simulink subsystem "rss_foc_controller_NewPlatform"  (R2023a)
settings: Solver=VariableStepAuto  StartTime=0.0  StopTime=10.0  RelTol=1e-3
undefined symbols (not defined in the file): Cdbl_tiFstTaskSmpTi, Cdbl_tiMedTaskSmpTi, Cdbl_tiSlwTaskSmpTi, ENM_AG_POS_EVAL_MODE, ENM_MOTO_STATUS, ENM_SYS_STATUS
(part 2 of 2)

== system rss_foc_controller_NewPlatform/vrs_DcycGenFstTaskIn/sss_DcycGenFstTaskInSenl ==
  u16_ampDycAmp : Inport
  u16_phiActElecAg : Inport  Port=2
  u16_phiDaxQaxVltgAg : Inport  Port=3
  enm_stMotoSt : Inport  Port=4
  s16_nPredActElecSpd : Inport  Port=5
  Bus Creator : BusCreator  Inputs=5  OutDataTypeStr=Bus: BUS_DCYCGEN_FST_TASK_IN
      settings: InheritFromInputs=off
  busDcycGen_FstTaskIn : Outport
  wires:
  Bus Creator/1 -> busDcycGen_FstTaskIn/1
  u16_ampDycAmp/1 -> Bus Creator/1
  u16_phiDaxQaxVltgAg/1 -> Bus Creator/3
  u16_phiActElecAg/1 -> Bus Creator/2
  s16_nPredActElecSpd/1 -> Bus Creator/5
  enm_stMotoSt/1 -> Bus Creator/4

== system rss_foc_controller_NewPlatform/vrs_DcycGenFstTaskIn/sss_DcycGenFstTaskInSens ==
  u16_ampDycAmp : Inport
  u16_phiActElecAg : Inport  Port=2
  u16_phiDaxQaxVltgAg : Inport  Port=3
  enm_stMotoSt : Inport  Port=4
  s16_nPredActElecSpd : Inport  Port=5
  bol_enPosSCDCalibEnFlg : Inport  Port=6
  Bus Creator : BusCreator  Inputs=6  OutDataTypeStr=Bus: BUS_DCYCGEN_FST_TASK_IN
      settings: InheritFromInputs=off
  busDcycGen_FstTaskIn : Outport
  wires:
  Bus Creator/1 -> busDcycGen_FstTaskIn/1
  bol_enPosSCDCalibEnFlg/1 -> Bus Creator/6
  u16_ampDycAmp/1 -> Bus Creator/1
  u16_phiDaxQaxVltgAg/1 -> Bus Creator/3
  u16_phiActElecAg/1 -> Bus Creator/2
  s16_nPredActElecSpd/1 -> Bus Creator/5
  enm_stMotoSt/1 -> Bus Creator/4

== system rss_foc_controller_NewPlatform/vrs_DcycGenFstTaskOut/sss_DcycGenFstTaskOutSenl ==
  busDcycGen_FstTaskOut : Inport
  Bus Selector1 : BusSelector  OutputSignals=u16_dcycPhDyc,u16_ampMaxNrmVltgAmp,u16_phiModulActElecAg
  u16_dcycPhDyc : Outport
  u16_ampMaxNrmVltgAmp : Outport  Port=2
  u16_phiModulActElecAg : Outport  Port=3
  wires:
  Bus Selector1/3 -> u16_phiModulActElecAg/1  "<u16_phiModulActElecAg>"
  Bus Selector1/1 -> u16_dcycPhDyc/1  "<u16_dcycPhDyc>"
  busDcycGen_FstTaskOut/1 -> Bus Selector1/1
  Bus Selector1/2 -> u16_ampMaxNrmVltgAmp/1  "<u16_ampMaxNrmVltgAmp>"

== system rss_foc_controller_NewPlatform/vrs_DcycGenFstTaskOut/sss_DcycGenFstTaskOutSens ==
  busDcycGen_FstTaskOut : Inport
  Bus Selector1 : BusSelector  OutputSignals=u16_dcycPhDyc,u16_ampMaxNrmVltgAmp,u16_phiModulActElecAg
  u16_dcycPhDyc : Outport
  u16_ampMaxNrmVltgAmp : Outport  Port=2
  u16_phiModulActElecAg : Outport  Port=3
  wires:
  Bus Selector1/3 -> u16_phiModulActElecAg/1  "<u16_phiModulActElecAg>"
  Bus Selector1/1 -> u16_dcycPhDyc/1  "<u16_dcycPhDyc>"
  busDcycGen_FstTaskOut/1 -> Bus Selector1/1
  Bus Selector1/2 -> u16_ampMaxNrmVltgAmp/1  "<u16_ampMaxNrmVltgAmp>"

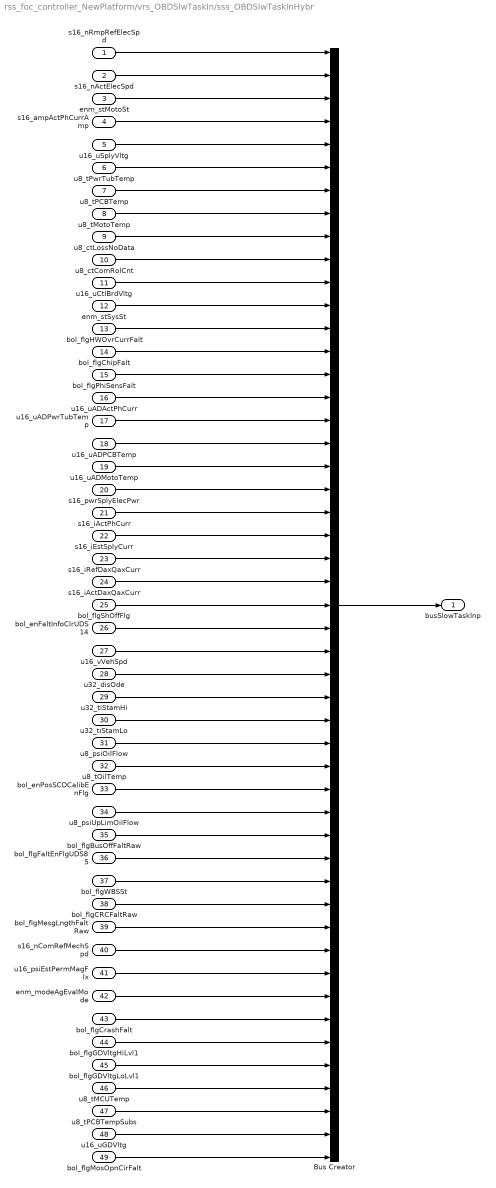
== system rss_foc_controller_NewPlatform/vrs_OBDSlwTaskIn/sss_OBDSlwTaskInHybr ==
  s16_nRmpRefElecSpd : Inport
  s16_nActElecSpd : Inport  Port=2
  enm_stMotoSt : Inport  Port=3
  s16_ampActPhCurrAmp : Inport  Port=4
  u16_uSplyVltg : Inport  Port=5
  u8_tPwrTubTemp : Inport  Port=6
  u8_tPCBTemp : Inport  Port=7
  u8_tMotoTemp : Inport  Port=8
  u8_ctLossNoData : Inport  Port=9
  u8_ctComRolCnt : Inport  Port=10
  u16_uCtlBrdVltg : Inport  Port=11
  enm_stSysSt : Inport  Port=12
  bol_flgHWOvrCurrFalt : Inport  Port=13
  bol_flgChipFalt : Inport  Port=14
  bol_flgPhiSensFalt : Inport  Port=15
  u16_uADActPhCurr : Inport  Port=16
  u16_uADPwrTubTemp : Inport  Port=17
  u16_uADPCBTemp : Inport  Port=18
  u16_uADMotoTemp : Inport  Port=19
  s16_pwrSplyElecPwr : Inport  Port=20
  s16_iActPhCurr : Inport  Port=21
  s16_iEstSplyCurr : Inport  Port=22
  s16_iRefDaxQaxCurr : Inport  Port=23
  s16_iActDaxQaxCurr : Inport  Port=24
  bol_flgShOffFlg : Inport  Port=25
  bol_enFaltInfoClrUDS14 : Inport  Port=26
  u16_vVehSpd : Inport  Port=27
  u32_disOde : Inport  Port=28
  u32_tiStamHi : Inport  Port=29
  u32_tiStamLo : Inport  Port=30
  u8_psiOilFlow : Inport  Port=31
  u8_tOilTemp : Inport  Port=32
  bol_enPosSCDCalibEnFlg : Inport  Port=33
  u8_psiUpLimOilFlow : Inport  Port=34
  bol_flgBusOffFaltRaw : Inport  Port=35
  bol_flgFaltEnFlgUDS85 : Inport  Port=36
  bol_flgWBSSt : Inport  Port=37
  bol_flgCRCFaltRaw : Inport  Port=38
  bol_flgMesgLngthFaltRaw : Inport  Port=39
  s16_nComRefMechSpd : Inport  Port=40
  u16_psiEstPermMagFlx : Inport  Port=41
  enm_modeAgEvalMode : Inport  Port=42
  bol_flgCrashFalt : Inport  Port=43
  bol_flgGDVltgHiLvl1 : Inport  Port=44
  bol_flgGDVltgLoLvl1 : Inport  Port=45
  u8_tMCUTemp : Inport  Port=46
  u8_tPCBTempSubs : Inport  Port=47
  u16_uGDVltg : Inport  Port=48
  bol_flgMosOpnCirFalt : Inport  Port=49
  Bus Creator : BusCreator  Inputs=49  OutDataTypeStr=Bus: BUS_OBD_SLW_TASK_IN
      settings: InheritFromInputs=off
  busSlowTaskInp : Outport  OutDataTypeStr=Bus: BUS_OBD_SLW_TASK_IN
  wires:
  bol_flgMosOpnCirFalt/1 -> Bus Creator/49
  u16_uGDVltg/1 -> Bus Creator/48
  u8_tPCBTempSubs/1 -> Bus Creator/47
  u8_tMCUTemp/1 -> Bus Creator/46
  bol_flgGDVltgLoLvl1/1 -> Bus Creator/45
  bol_flgGDVltgHiLvl1/1 -> Bus Creator/44
  bol_flgChipFalt/1 -> Bus Creator/14
  bol_flgCrashFalt/1 -> Bus Creator/43
  enm_modeAgEvalMode/1 -> Bus Creator/42
  bol_flgFaltEnFlgUDS85/1 -> Bus Creator/36
  s16_nRmpRefElecSpd/1 -> Bus Creator/1
  s16_nActElecSpd/1 -> Bus Creator/2
  enm_stMotoSt/1 -> Bus Creator/3
  s16_ampActPhCurrAmp/1 -> Bus Creator/4
  u16_uSplyVltg/1 -> Bus Creator/5
  u8_tPwrTubTemp/1 -> Bus Creator/6
  u8_tPCBTemp/1 -> Bus Creator/7
  u8_tMotoTemp/1 -> Bus Creator/8
  u8_ctLossNoData/1 -> Bus Creator/9
  u8_ctComRolCnt/1 -> Bus Creator/10
  Bus Creator/1 -> busSlowTaskInp/1
  u16_uCtlBrdVltg/1 -> Bus Creator/11
  enm_stSysSt/1 -> Bus Creator/12
  bol_flgHWOvrCurrFalt/1 -> Bus Creator/13
  bol_flgPhiSensFalt/1 -> Bus Creator/15
  u16_psiEstPermMagFlx/1 -> Bus Creator/41
  u16_uADActPhCurr/1 -> Bus Creator/16
  u16_uADPwrTubTemp/1 -> Bus Creator/17
  s16_nComRefMechSpd/1 -> Bus Creator/40
  bol_flgMesgLngthFaltRaw/1 -> Bus Creator/39
  bol_flgCRCFaltRaw/1 -> Bus Creator/38
  bol_flgWBSSt/1 -> Bus Creator/37
  bol_flgBusOffFaltRaw/1 -> Bus Creator/35
  u8_psiUpLimOilFlow/1 -> Bus Creator/34
  bol_enPosSCDCalibEnFlg/1 -> Bus Creator/33
  u8_tOilTemp/1 -> Bus Creator/32
  u8_psiOilFlow/1 -> Bus Creator/31
  u32_tiStamLo/1 -> Bus Creator/30
  u32_tiStamHi/1 -> Bus Creator/29
  u32_disOde/1 -> Bus Creator/28
  u16_vVehSpd/1 -> Bus Creator/27
  bol_enFaltInfoClrUDS14/1 -> Bus Creator/26
  bol_flgShOffFlg/1 -> Bus Creator/25
  s16_iActDaxQaxCurr/1 -> Bus Creator/24
  s16_iRefDaxQaxCurr/1 -> Bus Creator/23
  s16_iEstSplyCurr/1 -> Bus Creator/22
  s16_iActPhCurr/1 -> Bus Creator/21
  s16_pwrSplyElecPwr/1 -> Bus Creator/20
  u16_uADMotoTemp/1 -> Bus Creator/19
  u16_uADPCBTemp/1 -> Bus Creator/18

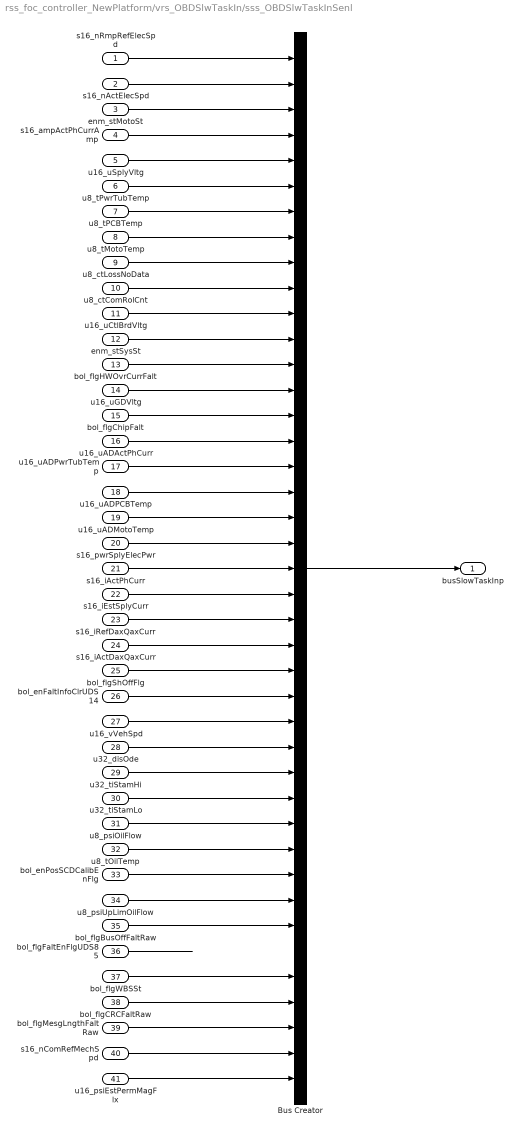
== system rss_foc_controller_NewPlatform/vrs_OBDSlwTaskIn/sss_OBDSlwTaskInSenl ==
  s16_nRmpRefElecSpd : Inport
  s16_nActElecSpd : Inport  Port=2
  enm_stMotoSt : Inport  Port=3
  s16_ampActPhCurrAmp : Inport  Port=4
  u16_uSplyVltg : Inport  Port=5
  u8_tPwrTubTemp : Inport  Port=6
  u8_tPCBTemp : Inport  Port=7
  u8_tMotoTemp : Inport  Port=8
  u8_ctLossNoData : Inport  Port=9
  u8_ctComRolCnt : Inport  Port=10
  u16_uCtlBrdVltg : Inport  Port=11
  enm_stSysSt : Inport  Port=12
  bol_flgHWOvrCurrFalt : Inport  Port=13
  u16_uGDVltg : Inport  Port=14
  bol_flgChipFalt : Inport  Port=15
  u16_uADActPhCurr : Inport  Port=16
  u16_uADPwrTubTemp : Inport  Port=17
  u16_uADPCBTemp : Inport  Port=18
  u16_uADMotoTemp : Inport  Port=19
  s16_pwrSplyElecPwr : Inport  Port=20
  s16_iActPhCurr : Inport  Port=21
  s16_iEstSplyCurr : Inport  Port=22
  s16_iRefDaxQaxCurr : Inport  Port=23
  s16_iActDaxQaxCurr : Inport  Port=24
  bol_flgShOffFlg : Inport  Port=25
  bol_enFaltInfoClrUDS14 : Inport  Port=26
  u16_vVehSpd : Inport  Port=27
  u32_disOde : Inport  Port=28
  u32_tiStamHi : Inport  Port=29
  u32_tiStamLo : Inport  Port=30
  u8_psiOilFlow : Inport  Port=31
  u8_tOilTemp : Inport  Port=32
  bol_enPosSCDCalibEnFlg : Inport  Port=33
  u8_psiUpLimOilFlow : Inport  Port=34
  bol_flgBusOffFaltRaw : Inport  Port=35
  bol_flgFaltEnFlgUDS85 : Inport  Port=36
  bol_flgWBSSt : Inport  Port=37
  bol_flgCRCFaltRaw : Inport  Port=38
  bol_flgMesgLngthFaltRaw : Inport  Port=39
  s16_nComRefMechSpd : Inport  Port=40
  u16_psiEstPermMagFlx : Inport  Port=41
  Bus Creator : BusCreator  Inputs=41  OutDataTypeStr=Bus: BUS_OBD_SLW_TASK_IN
      settings: InheritFromInputs=off
  busSlowTaskInp : Outport  OutDataTypeStr=Bus: BUS_OBD_SLW_TASK_IN
  wires:
  u16_uADPCBTemp/1 -> Bus Creator/18
  u16_uADMotoTemp/1 -> Bus Creator/19
  s16_pwrSplyElecPwr/1 -> Bus Creator/20
  s16_iActPhCurr/1 -> Bus Creator/21
  s16_iEstSplyCurr/1 -> Bus Creator/22
  s16_iRefDaxQaxCurr/1 -> Bus Creator/23
  s16_iActDaxQaxCurr/1 -> Bus Creator/24
  bol_flgShOffFlg/1 -> Bus Creator/25
  bol_enFaltInfoClrUDS14/1 -> Bus Creator/26
  u16_vVehSpd/1 -> Bus Creator/27
  u32_disOde/1 -> Bus Creator/28
  u32_tiStamHi/1 -> Bus Creator/29
  u32_tiStamLo/1 -> Bus Creator/30
  u8_psiOilFlow/1 -> Bus Creator/31
  u8_tOilTemp/1 -> Bus Creator/32
  bol_enPosSCDCalibEnFlg/1 -> Bus Creator/33
  u8_psiUpLimOilFlow/1 -> Bus Creator/34
  bol_flgBusOffFaltRaw/1 -> Bus Creator/35
  bol_flgFaltEnFlgUDS85/1 -> ?
  bol_flgWBSSt/1 -> Bus Creator/37
  bol_flgCRCFaltRaw/1 -> Bus Creator/38
  bol_flgMesgLngthFaltRaw/1 -> Bus Creator/39
  s16_nComRefMechSpd/1 -> Bus Creator/40
  u16_uADPwrTubTemp/1 -> Bus Creator/17
  u16_uADActPhCurr/1 -> Bus Creator/16
  u16_psiEstPermMagFlx/1 -> Bus Creator/41
  bol_flgChipFalt/1 -> Bus Creator/15
  u16_uGDVltg/1 -> Bus Creator/14
  bol_flgHWOvrCurrFalt/1 -> Bus Creator/13
  enm_stSysSt/1 -> Bus Creator/12
  u16_uCtlBrdVltg/1 -> Bus Creator/11
  Bus Creator/1 -> busSlowTaskInp/1
  u8_ctComRolCnt/1 -> Bus Creator/10
  u8_ctLossNoData/1 -> Bus Creator/9
  u8_tMotoTemp/1 -> Bus Creator/8
  u8_tPCBTemp/1 -> Bus Creator/7
  u8_tPwrTubTemp/1 -> Bus Creator/6
  u16_uSplyVltg/1 -> Bus Creator/5
  s16_ampActPhCurrAmp/1 -> Bus Creator/4
  enm_stMotoSt/1 -> Bus Creator/3
  s16_nActElecSpd/1 -> Bus Creator/2
  s16_nRmpRefElecSpd/1 -> Bus Creator/1

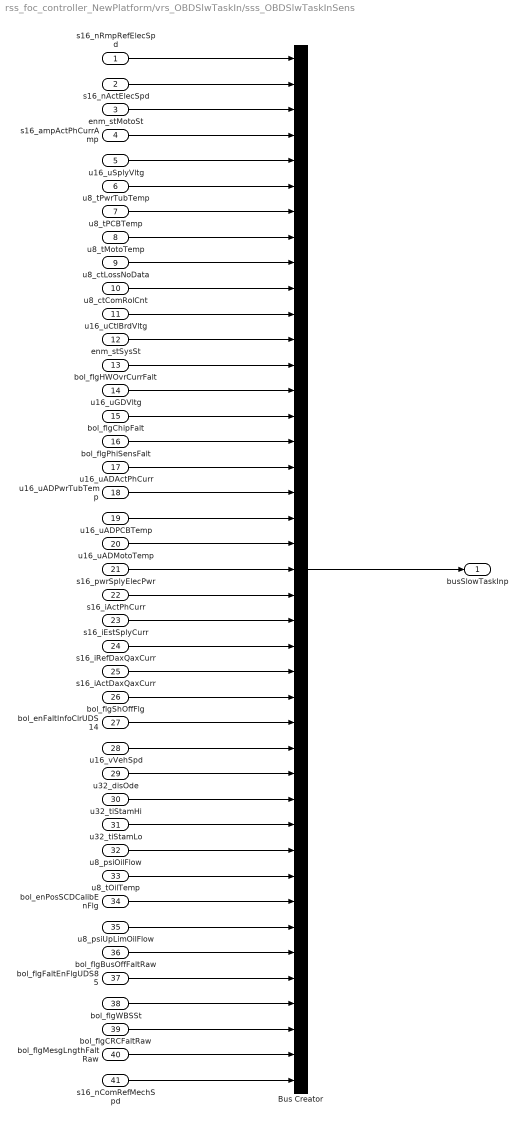
== system rss_foc_controller_NewPlatform/vrs_OBDSlwTaskIn/sss_OBDSlwTaskInSens ==
  s16_nRmpRefElecSpd : Inport
  s16_nActElecSpd : Inport  Port=2
  enm_stMotoSt : Inport  Port=3
  s16_ampActPhCurrAmp : Inport  Port=4
  u16_uSplyVltg : Inport  Port=5
  u8_tPwrTubTemp : Inport  Port=6
  u8_tPCBTemp : Inport  Port=7
  u8_tMotoTemp : Inport  Port=8
  u8_ctLossNoData : Inport  Port=9
  u8_ctComRolCnt : Inport  Port=10
  u16_uCtlBrdVltg : Inport  Port=11
  enm_stSysSt : Inport  Port=12
  bol_flgHWOvrCurrFalt : Inport  Port=13
  u16_uGDVltg : Inport  Port=14
  bol_flgChipFalt : Inport  Port=15
  bol_flgPhiSensFalt : Inport  Port=16
  u16_uADActPhCurr : Inport  Port=17
  u16_uADPwrTubTemp : Inport  Port=18
  u16_uADPCBTemp : Inport  Port=19
  u16_uADMotoTemp : Inport  Port=20
  s16_pwrSplyElecPwr : Inport  Port=21
  s16_iActPhCurr : Inport  Port=22
  s16_iEstSplyCurr : Inport  Port=23
  s16_iRefDaxQaxCurr : Inport  Port=24
  s16_iActDaxQaxCurr : Inport  Port=25
  bol_flgShOffFlg : Inport  Port=26
  bol_enFaltInfoClrUDS14 : Inport  Port=27
  u16_vVehSpd : Inport  Port=28
  u32_disOde : Inport  Port=29
  u32_tiStamHi : Inport  Port=30
  u32_tiStamLo : Inport  Port=31
  u8_psiOilFlow : Inport  Port=32
  u8_tOilTemp : Inport  Port=33
  bol_enPosSCDCalibEnFlg : Inport  Port=34
  u8_psiUpLimOilFlow : Inport  Port=35
  bol_flgBusOffFaltRaw : Inport  Port=36
  bol_flgFaltEnFlgUDS85 : Inport  Port=37
  bol_flgWBSSt : Inport  Port=38
  bol_flgCRCFaltRaw : Inport  Port=39
  bol_flgMesgLngthFaltRaw : Inport  Port=40
  s16_nComRefMechSpd : Inport  Port=41
  Bus Creator : BusCreator  Inputs=41  OutDataTypeStr=Bus: BUS_OBD_SLW_TASK_IN
      settings: InheritFromInputs=off
  busSlowTaskInp : Outport  OutDataTypeStr=Bus: BUS_OBD_SLW_TASK_IN
  wires:
  s16_nComRefMechSpd/1 -> Bus Creator/41
  bol_flgMesgLngthFaltRaw/1 -> Bus Creator/40
  bol_flgCRCFaltRaw/1 -> Bus Creator/39
  bol_flgWBSSt/1 -> Bus Creator/38
  bol_flgFaltEnFlgUDS85/1 -> Bus Creator/37
  bol_flgBusOffFaltRaw/1 -> Bus Creator/36
  u8_psiUpLimOilFlow/1 -> Bus Creator/35
  bol_enPosSCDCalibEnFlg/1 -> Bus Creator/34
  u8_tOilTemp/1 -> Bus Creator/33
  u8_psiOilFlow/1 -> Bus Creator/32
  u32_tiStamLo/1 -> Bus Creator/31
  u32_tiStamHi/1 -> Bus Creator/30
  u32_disOde/1 -> Bus Creator/29
  u16_vVehSpd/1 -> Bus Creator/28
  bol_enFaltInfoClrUDS14/1 -> Bus Creator/27
  bol_flgShOffFlg/1 -> Bus Creator/26
  s16_iActDaxQaxCurr/1 -> Bus Creator/25
  s16_iRefDaxQaxCurr/1 -> Bus Creator/24
  s16_iEstSplyCurr/1 -> Bus Creator/23
  s16_iActPhCurr/1 -> Bus Creator/22
  s16_pwrSplyElecPwr/1 -> Bus Creator/21
  u16_uADMotoTemp/1 -> Bus Creator/20
  u16_uADPCBTemp/1 -> Bus Creator/19
  u16_uADPwrTubTemp/1 -> Bus Creator/18
  u16_uADActPhCurr/1 -> Bus Creator/17
  bol_flgPhiSensFalt/1 -> Bus Creator/16
  bol_flgChipFalt/1 -> Bus Creator/15
  u16_uGDVltg/1 -> Bus Creator/14
  bol_flgHWOvrCurrFalt/1 -> Bus Creator/13
  enm_stSysSt/1 -> Bus Creator/12
  u16_uCtlBrdVltg/1 -> Bus Creator/11
  Bus Creator/1 -> busSlowTaskInp/1
  u8_ctComRolCnt/1 -> Bus Creator/10
  u8_ctLossNoData/1 -> Bus Creator/9
  u8_tMotoTemp/1 -> Bus Creator/8
  u8_tPCBTemp/1 -> Bus Creator/7
  u8_tPwrTubTemp/1 -> Bus Creator/6
  u16_uSplyVltg/1 -> Bus Creator/5
  s16_ampActPhCurrAmp/1 -> Bus Creator/4
  enm_stMotoSt/1 -> Bus Creator/3
  s16_nActElecSpd/1 -> Bus Creator/2
  s16_nRmpRefElecSpd/1 -> Bus Creator/1

== system rss_foc_controller_NewPlatform/vrs_OBDSlwTaskOut/sss_OBDSlwTaskOutHybr ==
  busOBD_SlwTaskOut : Inport
  Bus Selector2 : BusSelector  OutputSignals=busOBD_FaltSt,u8_stMaxFaltLvl,s16_nFaltRefMechSpd,s16_trqFaltRefTqLim,bol_flgPhiSensFaltRawFlg
  busOBD_FaltSt : Outport
  u8_stMaxFaltLvl : Outport  Port=2
  s16_nFaltRefMechSpd : Outport  Port=3
  s16_trqFaltRefTqLim : Outport  Port=4
  bol_flgPhiSensFaltRawFlg : Outport  Port=5
  wires:
  Bus Selector2/5 -> bol_flgPhiSensFaltRawFlg/1  "<bol_flgPhiSensFaltRawFlg>"
  Bus Selector2/2 -> u8_stMaxFaltLvl/1  "<u8_stMaxFaltLvl>"
  Bus Selector2/4 -> s16_trqFaltRefTqLim/1  "<s16_trqFaltRefTqLim>"
  busOBD_SlwTaskOut/1 -> Bus Selector2/1
  Bus Selector2/1 -> busOBD_FaltSt/1  "<busOBD_FaltSt>"
  Bus Selector2/3 -> s16_nFaltRefMechSpd/1  "<s16_nFaltRefMechSpd>"

== system rss_foc_controller_NewPlatform/vrs_OBDSlwTaskOut/sss_OBDSlwTaskOutSenl ==
  busOBD_SlwTaskOut : Inport
  Bus Selector2 : BusSelector  OutputSignals=busOBD_FaltSt,u8_stMaxFaltLvl,s16_nFaltRefMechSpd,s16_trqFaltRefTqLim
  busOBD_FaltSt : Outport
  u8_stMaxFaltLvl : Outport  Port=2
  s16_nFaltRefMechSpd : Outport  Port=3
  s16_trqFaltRefTqLim : Outport  Port=4
  wires:
  busOBD_SlwTaskOut/1 -> Bus Selector2/1
  Bus Selector2/1 -> busOBD_FaltSt/1  "<busOBD_FaltSt>"
  Bus Selector2/3 -> s16_nFaltRefMechSpd/1  "<s16_nFaltRefMechSpd>"
  Bus Selector2/2 -> u8_stMaxFaltLvl/1  "<u8_stMaxFaltLvl>"
  Bus Selector2/4 -> s16_trqFaltRefTqLim/1  "<s16_trqFaltRefTqLim>"

== system rss_foc_controller_NewPlatform/vrs_OBDSlwTaskOut/sss_OBDSlwTaskOutSens ==
  busOBD_SlwTaskOut : Inport
  Bus Selector2 : BusSelector  OutputSignals=busOBD_FaltSt,u8_stMaxFaltLvl,s16_nFaltRefMechSpd,s16_trqFaltRefTqLim
  busOBD_FaltSt : Outport
  u8_stMaxFaltLvl : Outport  Port=2
  s16_nFaltRefMechSpd : Outport  Port=3
  s16_trqFaltRefTqLim : Outport  Port=4
  wires:
  Bus Selector2/4 -> s16_trqFaltRefTqLim/1  "<s16_trqFaltRefTqLim>"
  Bus Selector2/3 -> s16_nFaltRefMechSpd/1  "<s16_nFaltRefMechSpd>"
  Bus Selector2/2 -> u8_stMaxFaltLvl/1  "<u8_stMaxFaltLvl>"
  Bus Selector2/1 -> busOBD_FaltSt/1  "<busOBD_FaltSt>"
  busOBD_SlwTaskOut/1 -> Bus Selector2/1

== system rss_foc_controller_NewPlatform/vrs_PhCurrGenSlwTaskIn/sss_PhCurrGenSlwTaskInHybr ==
  s16_nRefElecSpd : Inport
  s16_nActElecSpd : Inport  Port=2
  s16_nRmpRefElecSpd : Inport  Port=3
  s16_trqRefTqLim : Inport  Port=4
  bol_flgShOffFlg : Inport  Port=5
  bol_enPosSCDCalibEnFlg : Inport  Port=6
  s16_trqPosSCDCalibRefTq : Inport  Port=7
  enm_modeAgEvalMode : Inport  Port=8
  s16_phiOpnLpAgClsLpAgDvt : Inport  Port=9
  Bus Creator : BusCreator  Inputs=9  OutDataTypeStr=Bus: BUS_PHCURRGEN_SLW_TASK_IN
      settings: InheritFromInputs=off
  busPhCurrGen_SlwTaskIn : Outport  OutDataTypeStr=Bus: BUS_PHCURRGEN_SLW_TASK_IN
  wires:
  s16_phiOpnLpAgClsLpAgDvt/1 -> Bus Creator/9
  enm_modeAgEvalMode/1 -> Bus Creator/8
  s16_trqPosSCDCalibRefTq/1 -> Bus Creator/7
  bol_enPosSCDCalibEnFlg/1 -> Bus Creator/6
  s16_nRefElecSpd/1 -> Bus Creator/1
  s16_nActElecSpd/1 -> Bus Creator/2
  s16_nRmpRefElecSpd/1 -> Bus Creator/3
  s16_trqRefTqLim/1 -> Bus Creator/4
  bol_flgShOffFlg/1 -> Bus Creator/5
  Bus Creator/1 -> busPhCurrGen_SlwTaskIn/1

== system rss_foc_controller_NewPlatform/vrs_PhCurrGenSlwTaskIn/sss_PhCurrGenSlwTaskInSenl ==
  s16_nRefElecSpd : Inport
  s16_nActElecSpd : Inport  Port=2
  s16_nRmpRefElecSpd : Inport  Port=3
  s16_trqRefTqLim : Inport  Port=4
  bol_flgShOffFlg : Inport  Port=5
  Bus Creator : BusCreator  Inputs=5  OutDataTypeStr=Bus: BUS_PHCURRGEN_SLW_TASK_IN
      settings: InheritFromInputs=off
  busPhCurrGen_SlwTaskIn : Outport  OutDataTypeStr=Bus: BUS_PHCURRGEN_SLW_TASK_IN
  wires:
  Bus Creator/1 -> busPhCurrGen_SlwTaskIn/1
  bol_flgShOffFlg/1 -> Bus Creator/5
  s16_trqRefTqLim/1 -> Bus Creator/4
  s16_nRmpRefElecSpd/1 -> Bus Creator/3
  s16_nActElecSpd/1 -> Bus Creator/2
  s16_nRefElecSpd/1 -> Bus Creator/1

== system rss_foc_controller_NewPlatform/vrs_PhCurrGenSlwTaskIn/sss_PhCurrGenSlwTaskInSens ==
  s16_nRefElecSpd : Inport
  s16_nActElecSpd : Inport  Port=2
  s16_nRmpRefElecSpd : Inport  Port=3
  s16_trqRefTqLim : Inport  Port=4
  bol_flgShOffFlg : Inport  Port=5
  bol_enPosSCDCalibEnFlg : Inport  Port=6
  s16_trqPosSCDCalibRefTq : Inport  Port=7
  Bus Creator : BusCreator  Inputs=7  OutDataTypeStr=Bus: BUS_PHCURRGEN_SLW_TASK_IN
      settings: InheritFromInputs=off
  busPhCurrGen_SlwTaskIn : Outport  OutDataTypeStr=Bus: BUS_PHCURRGEN_SLW_TASK_IN
  wires:
  Bus Creator/1 -> busPhCurrGen_SlwTaskIn/1
  s16_trqPosSCDCalibRefTq/1 -> Bus Creator/7
  bol_enPosSCDCalibEnFlg/1 -> Bus Creator/6
  bol_flgShOffFlg/1 -> Bus Creator/5
  s16_trqRefTqLim/1 -> Bus Creator/4
  s16_nRmpRefElecSpd/1 -> Bus Creator/3
  s16_nActElecSpd/1 -> Bus Creator/2
  s16_nRefElecSpd/1 -> Bus Creator/1

== system rss_foc_controller_NewPlatform/vrs_PhCurrGenSlwTaskOut/sss_PhCurrGenSlwTaskOutHybr ==
  busMotoCtl_SlwTaskOut : Inport
  Bus Selector2 : BusSelector  OutputSignals=iRefDQCurr,iEstSplyCurr,iActLineCurr,bolDrtnFlag,bolStrtUpProcOk,wRefElctSpd,iCalibCurr,arCalibElecAng,bolCalibSuccFlag,arSensErrMechAng,AngSensCalib_Status,mtrAlgPermFail
  s16_iRefDaxQaxCurr : Outport
  iEstSplyCurr : Outport  Port=2
  iActLineCurr : Outport  Port=3
  bolDrtnFlag : Outport  Port=4
  bolStrtUpProcOk : Outport  Port=5
  wRefElctSpd : Outport  Port=6
  iCalibCurr : Outport  Port=7
  arCalibElecAng : Outport  Port=8
  bolCalibSuccFlag : Outport  Port=9
  arSensErrMechAng : Outport  Port=10
  AngSensCalib_Status : Outport  Port=11
  mtrAlgPermFail : Outport  Port=12
  wires:
  Bus Selector2/12 -> mtrAlgPermFail/1  "<mtrAlgPermFail>"
  Bus Selector2/11 -> AngSensCalib_Status/1  "<AngSensCalib_Status>"
  Bus Selector2/10 -> arSensErrMechAng/1  "<arSensErrMechAng>"
  Bus Selector2/9 -> bolCalibSuccFlag/1  "<bolCalibSuccFlag>"
  Bus Selector2/8 -> arCalibElecAng/1  "<arCalibElecAng>"
  Bus Selector2/7 -> iCalibCurr/1  "<iCalibCurr>"
  busMotoCtl_SlwTaskOut/1 -> Bus Selector2/1
  Bus Selector2/5 -> bolStrtUpProcOk/1  "<bolStrtUpProcOk>"
  Bus Selector2/1 -> s16_iRefDaxQaxCurr/1  "<iRefDQCurr>"
  Bus Selector2/4 -> bolDrtnFlag/1  "<bolDrtnFlag>"
  Bus Selector2/6 -> wRefElctSpd/1  "<wRefElctSpd>"
  Bus Selector2/2 -> iEstSplyCurr/1  "<iEstSplyCurr>"
  Bus Selector2/3 -> iActLineCurr/1  "<iActLineCurr>"

== system rss_foc_controller_NewPlatform/vrs_PhCurrGenSlwTaskOut/sss_PhCurrGenSlwTaskOutSenl ==
  busMotoCtl_SlwTaskOut : Inport
  Bus Selector2 : BusSelector  OutputSignals=s16_iRefDaxQaxCurr,enm_stMotoSt
  s16_iRefDaxQaxCurr : Outport
  enm_stMotoSt : Outport  Port=2
  wires:
  Bus Selector2/1 -> s16_iRefDaxQaxCurr/1  "<s16_iRefDaxQaxCurr>"
  busMotoCtl_SlwTaskOut/1 -> Bus Selector2/1
  Bus Selector2/2 -> enm_stMotoSt/1  "<enm_stMotoSt>"

== system rss_foc_controller_NewPlatform/vrs_PhCurrGenSlwTaskOut/sss_PhCurrGenSlwTaskOutSens ==
  busMotoCtl_SlwTaskOut : Inport
  Bus Selector2 : BusSelector  OutputSignals=s16_iRefDaxQaxCurr,enm_stMotoSt
  s16_iRefDaxQaxCurr : Outport
  enm_stMotoSt : Outport  Port=2
  wires:
  Bus Selector2/2 -> enm_stMotoSt/1  "<enm_stMotoSt>"
  busMotoCtl_SlwTaskOut/1 -> Bus Selector2/1
  Bus Selector2/1 -> s16_iRefDaxQaxCurr/1  "<s16_iRefDaxQaxCurr>"

== system rss_foc_controller_NewPlatform/vrs_PhVltgGenMedTaskIn/sss_PhVltgGenMedTaskInHybr ==
  s16_iRefDaxQaxCurr : Inport
  s16_iActPhCurr : Inport  Port=2
  u16_phiSensActElecAg : Inport  Port=3
  u16_uSplyVltg : Inport  Port=4
  enm_stMotoSt : Inport  Port=5
  u16_phiModulActElecAg : Inport  Port=6
  u16_phiPosSCDCalibElecAg : Inport  Port=7
  u16_dcycPhDyc : Inport  Port=8
  bol_enPosSCDCalibEnFlg : Inport  Port=9
  enm_modeAgEvalMode : Inport  Port=10
  s16_nRmpRefElecSpd : Inport  Port=11
  u8_tPCBTempSubs : Inport  Port=12
  u16_ampMaxNrmVltgAmp : Inport  Port=13
  Bus Creator1 : BusCreator  Inputs=13  OutDataTypeStr=Bus: BUS_PHVLTGGEN_MED_TASK_IN
      settings: InheritFromInputs=off
  busPhVltgGen_MedTaskIn : Outport
  wires:
  u16_ampMaxNrmVltgAmp/1 -> Bus Creator1/13
  u8_tPCBTempSubs/1 -> Bus Creator1/12
  u16_phiModulActElecAg/1 -> Bus Creator1/6
  u16_uSplyVltg/1 -> Bus Creator1/4
  s16_iRefDaxQaxCurr/1 -> Bus Creator1/1
  u16_dcycPhDyc/1 -> Bus Creator1/8
  u16_phiSensActElecAg/1 -> Bus Creator1/3
  enm_modeAgEvalMode/1 -> Bus Creator1/10
  enm_stMotoSt/1 -> Bus Creator1/5
  Bus Creator1/1 -> busPhVltgGen_MedTaskIn/1
  s16_nRmpRefElecSpd/1 -> Bus Creator1/11
  u16_phiPosSCDCalibElecAg/1 -> Bus Creator1/7
  bol_enPosSCDCalibEnFlg/1 -> Bus Creator1/9
  s16_iActPhCurr/1 -> Bus Creator1/2

== system rss_foc_controller_NewPlatform/vrs_PhVltgGenMedTaskIn/sss_PhVltgGenMedTaskInSenl ==
  s16_iRefDaxQaxCurr : Inport
  s16_iActPhCurr : Inport  Port=2
  u16_phiSensActElecAg : Inport  Port=3
  u16_uSplyVltg : Inport  Port=4
  enm_stMotoSt : Inport  Port=5
  u16_phiModulActElecAg : Inport  Port=6
  u16_dcycPhDyc : Inport  Port=7
  s16_nRmpRefElecSpd : Inport  Port=8
  u16_ampMaxVltgAmp : Inport  Port=9
  s16_uRefDaxVltgLim : Inport  Port=10
  s16_uRefQaxVltgLim : Inport  Port=11
  Bus Creator1 : BusCreator  Inputs=11  OutDataTypeStr=Bus: BUS_PHVLTGGEN_MED_TASK_IN
      settings: InheritFromInputs=off
  busPhVltgGen_MedTaskIn : Outport
  wires:
  Bus Creator1/1 -> busPhVltgGen_MedTaskIn/1
  s16_uRefQaxVltgLim/1 -> Bus Creator1/11
  s16_uRefDaxVltgLim/1 -> Bus Creator1/10
  u16_ampMaxVltgAmp/1 -> Bus Creator1/9
  s16_nRmpRefElecSpd/1 -> Bus Creator1/8
  u16_dcycPhDyc/1 -> Bus Creator1/7
  u16_phiModulActElecAg/1 -> Bus Creator1/6
  enm_stMotoSt/1 -> Bus Creator1/5
  u16_uSplyVltg/1 -> Bus Creator1/4
  u16_phiSensActElecAg/1 -> Bus Creator1/3
  s16_iRefDaxQaxCurr/1 -> Bus Creator1/1
  s16_iActPhCurr/1 -> Bus Creator1/2

== system rss_foc_controller_NewPlatform/vrs_PhVltgGenMedTaskIn/sss_PhVltgGenMedTaskInSens ==
  s16_iRefDaxQaxCurr : Inport
  s16_iActPhCurr : Inport  Port=2
  u16_phiSensActElecAg : Inport  Port=3
  u16_uSplyVltg : Inport  Port=4
  enm_stMotoSt : Inport  Port=5
  u16_phiModulActElecAg : Inport  Port=6
  u16_phiPosSCDCalibElecAg : Inport  Port=7  OutDataTypeStr=dt_RadAng_u16r15b0
  u16_dcycPhDyc : Inport  Port=8
  bol_enPosSCDCalibEnFlg : Inport  Port=9
  s16_nRmpRefElecSpd : Inport  Port=10
  u16_ampMaxVltgAmp : Inport  Port=11
  s16_uRefDaxVltgLim : Inport  Port=12
  s16_uRefQaxVltgLim : Inport  Port=13
  Bus Creator1 : BusCreator  Inputs=13  OutDataTypeStr=Bus: BUS_PHVLTGGEN_MED_TASK_IN
      settings: InheritFromInputs=off
  busPhVltgGen_MedTaskIn : Outport
  wires:
  Bus Creator1/1 -> busPhVltgGen_MedTaskIn/1
  s16_uRefQaxVltgLim/1 -> Bus Creator1/13
  s16_uRefDaxVltgLim/1 -> Bus Creator1/12
  u16_ampMaxVltgAmp/1 -> Bus Creator1/11
  s16_nRmpRefElecSpd/1 -> Bus Creator1/10
  bol_enPosSCDCalibEnFlg/1 -> Bus Creator1/9
  u16_dcycPhDyc/1 -> Bus Creator1/8
  u16_phiPosSCDCalibElecAg/1 -> Bus Creator1/7
  u16_phiModulActElecAg/1 -> Bus Creator1/6
  s16_iActPhCurr/1 -> Bus Creator1/2
  enm_stMotoSt/1 -> Bus Creator1/5
  u16_uSplyVltg/1 -> Bus Creator1/4
  s16_iRefDaxQaxCurr/1 -> Bus Creator1/1
  u16_phiSensActElecAg/1 -> Bus Creator1/3

== system rss_foc_controller_NewPlatform/vrs_PhVltgGenMedTaskOut/sss_PhVltgGenMedTaskOutHybr ==
  busPhVltgGen_MedTaskOut : Inport
  Bus Selector : BusSelector  OutputSignals=u16_ampDycAmp,u16_phiDaxQaxVltgAg,u16_phiActElecAg,s16_nActElecSpd,s16_iActDaxQaxCurr,s16_nPredActElecSpd,s16_uModulDaxQaxVltg,u16_psiEstPermMagFlx,s16_phiOpnLpAgClsLpAgDvt
  u16_ampDycAmp : Outport
  u16_phiDaxQaxVltgAg : Outport  Port=2
  u16_phiActElecAg : Outport  Port=3
  s16_nActElecSpd : Outport  Port=4
  s16_iActDaxQaxCurr : Outport  Port=5
  s16_nPredActElecSpd : Outport  Port=6
  s16_uModulDaxQaxVltg : Outport  Port=7
  u16_psiEstPermMagFlx : Outport  Port=8
  s16_phiOpnLpAgClsLpAgDvt : Outport  Port=9
  wires:
  Bus Selector/9 -> s16_phiOpnLpAgClsLpAgDvt/1  "<s16_phiOpnLpAgClsLpAgDvt>"
  busPhVltgGen_MedTaskOut/1 -> Bus Selector/1
  Bus Selector/5 -> s16_iActDaxQaxCurr/1  "<s16_iActDaxQaxCurr>"
  Bus Selector/1 -> u16_ampDycAmp/1  "<u16_ampDycAmp>"
  Bus Selector/4 -> s16_nActElecSpd/1  "<s16_nActElecSpd>"
  Bus Selector/7 -> s16_uModulDaxQaxVltg/1  "<s16_uModulDaxQaxVltg>"
  Bus Selector/3 -> u16_phiActElecAg/1  "<u16_phiActElecAg>"
  Bus Selector/6 -> s16_nPredActElecSpd/1  "<s16_nPredActElecSpd>"
  Bus Selector/2 -> u16_phiDaxQaxVltgAg/1  "<u16_phiDaxQaxVltgAg>"
  Bus Selector/8 -> u16_psiEstPermMagFlx/1  "<u16_psiEstPermMagFlx>"

== system rss_foc_controller_NewPlatform/vrs_PhVltgGenMedTaskOut/sss_PhVltgGenMedTaskOutSenl ==
  busPhVltgGen_MedTaskOut : Inport
  Bus Selector : BusSelector  OutputSignals=u16_ampDycAmp,u16_phiDaxQaxVltgAg,u16_phiActElecAg,s16_nActElecSpd,s16_iActDaxQaxCurr,s16_nPredActElecSpd,s16_uModulDaxQaxVltg,s16_uRefDaxVltg,u16_psiEstPermMagFlx
  u16_ampDycAmp : Outport
  u16_phiDaxQaxVltgAg : Outport  Port=2
  u16_phiActElecAg : Outport  Port=3
  s16_nActElecSpd : Outport  Port=4
  s16_iActDaxQaxCurr : Outport  Port=5
  s16_nPredActElecSpd : Outport  Port=6
  s16_uModulDaxQaxVltg : Outport  Port=7
  s16_uRefDaxVltg : Outport  Port=8
  u16_psiEstPermMagFlx : Outport  Port=9
  wires:
  Bus Selector/9 -> u16_psiEstPermMagFlx/1  "<u16_psiEstPermMagFlx>"
  Bus Selector/8 -> s16_uRefDaxVltg/1  "<s16_uRefDaxVltg>"
  Bus Selector/2 -> u16_phiDaxQaxVltgAg/1  "<u16_phiDaxQaxVltgAg>"
  Bus Selector/6 -> s16_nPredActElecSpd/1  "<s16_nPredActElecSpd>"
  busPhVltgGen_MedTaskOut/1 -> Bus Selector/1
  Bus Selector/1 -> u16_ampDycAmp/1  "<u16_ampDycAmp>"
  Bus Selector/4 -> s16_nActElecSpd/1  "<s16_nActElecSpd>"
  Bus Selector/3 -> u16_phiActElecAg/1  "<u16_phiActElecAg>"
  Bus Selector/7 -> s16_uModulDaxQaxVltg/1  "<s16_uModulDaxQaxVltg>"
  Bus Selector/5 -> s16_iActDaxQaxCurr/1  "<s16_iActDaxQaxCurr>"

== system rss_foc_controller_NewPlatform/vrs_PhVltgGenMedTaskOut/sss_PhVltgGenMedTaskOutSens ==
  busPhVltgGen_MedTaskOut : Inport
  Bus Selector : BusSelector  OutputSignals=u16_ampDycAmp,u16_phiDaxQaxVltgAg,u16_phiActElecAg,s16_nActElecSpd,s16_iActDaxQaxCurr,s16_nPredActElecSpd,s16_uModulDaxQaxVltg,s16_uRefDaxVltg
  u16_ampDycAmp : Outport
  u16_phiDaxQaxVltgAg : Outport  Port=2
  u16_phiActElecAg : Outport  Port=3
  s16_nActElecSpd : Outport  Port=4
  s16_iActDaxQaxCurr : Outport  Port=5
  s16_nPredActElecSpd : Outport  Port=6
  s16_uModulDaxQaxVltg : Outport  Port=7
  s16_uRefDaxVltg : Outport  Port=8
  wires:
  Bus Selector/8 -> s16_uRefDaxVltg/1  "<s16_uRefDaxVltg>"
  Bus Selector/2 -> u16_phiDaxQaxVltgAg/1  "<u16_phiDaxQaxVltgAg>"
  Bus Selector/6 -> s16_nPredActElecSpd/1  "<s16_nPredActElecSpd>"
  busPhVltgGen_MedTaskOut/1 -> Bus Selector/1
  Bus Selector/1 -> u16_ampDycAmp/1  "<u16_ampDycAmp>"
  Bus Selector/4 -> s16_nActElecSpd/1  "<s16_nActElecSpd>"
  Bus Selector/3 -> u16_phiActElecAg/1  "<u16_phiActElecAg>"
  Bus Selector/7 -> s16_uModulDaxQaxVltg/1  "<s16_uModulDaxQaxVltg>"
  Bus Selector/5 -> s16_iActDaxQaxCurr/1  "<s16_iActDaxQaxCurr>"

== system rss_foc_controller_NewPlatform/vrs_SigInMedTaskIn/sss_SigInMedTaskInSenl ==
  u16_uADActPhCurr : Inport
  u16_uADActPhCurrOfs : Inport  Port=2
  u8_numSectNum : Inport  Port=3
  Bus Creator : BusCreator  Inputs=3  OutDataTypeStr=Bus: BUS_SIGIN_MED_TASK_IN
      settings: InheritFromInputs=off
  busSigIn_MedTaskIn : Outport  OutDataTypeStr=Bus: BUS_SIGIN_MED_TASK_IN
  wires:
  u16_uADActPhCurr/1 -> Bus Creator/1
  u16_uADActPhCurrOfs/1 -> Bus Creator/2
  Bus Creator/1 -> busSigIn_MedTaskIn/1
  u8_numSectNum/1 -> Bus Creator/3

== system rss_foc_controller_NewPlatform/vrs_SigInMedTaskIn/sss_SigInMedTaskInSens ==
  u16_ADSensActMechAg : Inport
  u16_uADActPhCurr : Inport  Port=2
  u16_uADActPhCurrOfs : Inport  Port=3
  u8_numSectNum : Inport  Port=4
  u16_uADSplyVltg : Inport  Port=5
  u16_phiDvtSensElecAg : Inport  Port=6
  bol_enPosSCDCalibEnFlg : Inport  Port=7
  Bus Creator : BusCreator  Inputs=7  OutDataTypeStr=Bus: BUS_SIGIN_MED_TASK_IN
      settings: InheritFromInputs=off
  busSigIn_MedTaskIn : Outport  OutDataTypeStr=Bus: BUS_SIGIN_MED_TASK_IN
  wires:
  bol_enPosSCDCalibEnFlg/1 -> Bus Creator/7
  u16_phiDvtSensElecAg/1 -> Bus Creator/6
  u16_uADSplyVltg/1 -> Bus Creator/5
  Bus Creator/1 -> busSigIn_MedTaskIn/1
  u8_numSectNum/1 -> Bus Creator/4
  u16_uADActPhCurrOfs/1 -> Bus Creator/3
  u16_uADActPhCurr/1 -> Bus Creator/2
  u16_ADSensActMechAg/1 -> Bus Creator/1

== system rss_foc_controller_NewPlatform/vrs_SigInMedTaskOut/sss_SigInMedTaskOutHybr ==
  busSigIn_MedTaskOut : Inport
  Bus Selector2 : BusSelector  OutputSignals=iRefDQCurr,iEstSplyCurr,iActLineCurr,bolDrtnFlag,bolStrtUpProcOk,wRefElctSpd,iCalibCurr,arCalibElecAng,bolCalibSuccFlag,arSensErrMechAng,AngSensCalib_Status,mtrAlgPermFail
  iRefDQCurr : Outport
  iEstSplyCurr : Outport  Port=2
  iActLineCurr : Outport  Port=3
  u16_phiSensActElecAg : Outport  Port=4
  bolStrtUpProcOk : Outport  Port=5
  wRefElctSpd : Outport  Port=6
  iCalibCurr : Outport  Port=7
  arCalibElecAng : Outport  Port=8
  bolCalibSuccFlag : Outport  Port=9
  arSensErrMechAng : Outport  Port=10
  AngSensCalib_Status : Outport  Port=11
  mtrAlgPermFail : Outport  Port=12
  wires:
  Bus Selector2/12 -> mtrAlgPermFail/1  "<mtrAlgPermFail>"
  Bus Selector2/11 -> AngSensCalib_Status/1  "<AngSensCalib_Status>"
  Bus Selector2/10 -> arSensErrMechAng/1  "<arSensErrMechAng>"
  Bus Selector2/9 -> bolCalibSuccFlag/1  "<bolCalibSuccFlag>"
  Bus Selector2/8 -> arCalibElecAng/1  "<arCalibElecAng>"
  Bus Selector2/7 -> iCalibCurr/1  "<iCalibCurr>"
  busSigIn_MedTaskOut/1 -> Bus Selector2/1
  Bus Selector2/5 -> bolStrtUpProcOk/1  "<bolStrtUpProcOk>"
  Bus Selector2/1 -> iRefDQCurr/1  "<iRefDQCurr>"
  Bus Selector2/4 -> u16_phiSensActElecAg/1  "<bolDrtnFlag>"
  Bus Selector2/6 -> wRefElctSpd/1  "<wRefElctSpd>"
  Bus Selector2/2 -> iEstSplyCurr/1  "<iEstSplyCurr>"
  Bus Selector2/3 -> iActLineCurr/1  "<iActLineCurr>"

== system rss_foc_controller_NewPlatform/vrs_SigInMedTaskOut/sss_SigInMedTaskOutSenl ==
  busSigIn_MedTaskOut : Inport
  Bus Selector2 : BusSelector  OutputSignals=s16_iActPhCurr
  s16_iActPhCurr : Outport
  wires:
  busSigIn_MedTaskOut/1 -> Bus Selector2/1
  Bus Selector2/1 -> s16_iActPhCurr/1  "<s16_iActPhCurr>"

== system rss_foc_controller_NewPlatform/vrs_SigInMedTaskOut/sss_SigInMedTaskOutSens ==
  busSigIn_MedTaskOut : Inport
  Bus Selector2 : BusSelector  OutputSignals=u16_phiSensActElecAg,s16_iActPhCurr,u16_uSplyVltg
  u16_phiSensActElecAg : Outport
  s16_iActPhCurr : Outport  Port=2
  u16_uSplyVltg : Outport  Port=3
  wires:
  Bus Selector2/3 -> u16_uSplyVltg/1  "<u16_uSplyVltg>"
  Bus Selector2/2 -> s16_iActPhCurr/1  "<s16_iActPhCurr>"
  busSigIn_MedTaskOut/1 -> Bus Selector2/1
  Bus Selector2/1 -> u16_phiSensActElecAg/1  "<u16_phiSensActElecAg>"

== system rss_foc_controller_NewPlatform/vrs_SigInSlwTaskOut/sss_SigInSlwTaskOutHybr ==
  busSigIn_SlwTaskOut : Inport
  Bus Selector2 : BusSelector  OutputSignals=iRefDQCurr,iEstSplyCurr,iActLineCurr,bolDrtnFlag,bolStrtUpProcOk,wRefElctSpd,iCalibCurr,arCalibElecAng,bolCalibSuccFlag,arSensErrMechAng,AngSensCalib_Status,mtrAlgPermFail
  iRefDQCurr : Outport
  iEstSplyCurr : Outport  Port=2
  iActLineCurr : Outport  Port=3
  arSensActElctAng : Outport  Port=4
  bolStrtUpProcOk : Outport  Port=5
  wRefElctSpd : Outport  Port=6
  iCalibCurr : Outport  Port=7
  arCalibElecAng : Outport  Port=8
  bolCalibSuccFlag : Outport  Port=9
  arSensErrMechAng : Outport  Port=10
  AngSensCalib_Status : Outport  Port=11
  mtrAlgPermFail : Outport  Port=12
  wires:
  Bus Selector2/3 -> iActLineCurr/1  "<iActLineCurr>"
  Bus Selector2/2 -> iEstSplyCurr/1  "<iEstSplyCurr>"
  Bus Selector2/6 -> wRefElctSpd/1  "<wRefElctSpd>"
  Bus Selector2/4 -> arSensActElctAng/1  "<bolDrtnFlag>"
  Bus Selector2/1 -> iRefDQCurr/1  "<iRefDQCurr>"
  Bus Selector2/5 -> bolStrtUpProcOk/1  "<bolStrtUpProcOk>"
  busSigIn_SlwTaskOut/1 -> Bus Selector2/1
  Bus Selector2/7 -> iCalibCurr/1  "<iCalibCurr>"
  Bus Selector2/8 -> arCalibElecAng/1  "<arCalibElecAng>"
  Bus Selector2/9 -> bolCalibSuccFlag/1  "<bolCalibSuccFlag>"
  Bus Selector2/10 -> arSensErrMechAng/1  "<arSensErrMechAng>"
  Bus Selector2/11 -> AngSensCalib_Status/1  "<AngSensCalib_Status>"
  Bus Selector2/12 -> mtrAlgPermFail/1  "<mtrAlgPermFail>"

== system rss_foc_controller_NewPlatform/vrs_SigInSlwTaskOut/sss_SigInSlwTaskOutSenl ==
  busSigIn_SlwTaskOut : Inport
  Bus Selector2 : BusSelector  OutputSignals=u16_uCtlBrdVltg,u16_uGDVltg,u8_tPwrTubTemp,u8_tPCBTemp,u8_tMotoTemp,u8_tPCBTempSubs
  u16_uCtlBrdVltg : Outport
  u16_uGDVltg : Outport  Port=2
  u8_tPwrTubTemp : Outport  Port=3
  u8_tPCBTemp : Outport  Port=4
  u8_tMotoTemp : Outport  Port=5
  u8_tPCBTempSubs : Outport  Port=6
  wires:
  Bus Selector2/6 -> u8_tPCBTempSubs/1  "<u8_tPCBTempSubs>"
  Bus Selector2/2 -> u16_uGDVltg/1  "<u16_uGDVltg>"
  Bus Selector2/1 -> u16_uCtlBrdVltg/1  "<u16_uCtlBrdVltg>"
  busSigIn_SlwTaskOut/1 -> Bus Selector2/1
  Bus Selector2/5 -> u8_tMotoTemp/1  "<u8_tMotoTemp>"
  Bus Selector2/4 -> u8_tPCBTemp/1  "<u8_tPCBTemp>"
  Bus Selector2/3 -> u8_tPwrTubTemp/1  "<u8_tPwrTubTemp>"

== system rss_foc_controller_NewPlatform/vrs_SigInSlwTaskOut/sss_SigInSlwTaskOutSens ==
  busSigIn_SlwTaskOut : Inport
  Bus Selector2 : BusSelector  OutputSignals=u16_uSplyVltg,u16_uCtlBrdVltg,u16_uGDVltg,u8_tPwrTubTemp,u8_tPCBTemp,u8_tMotoTemp
  u16_uSplyVltg : Outport
  u16_uCtlBrdVltg : Outport  Port=2
  u16_uGDVltg : Outport  Port=3
  u8_tPwrTubTemp : Outport  Port=4
  u8_tPCBTemp : Outport  Port=5
  u8_tMotoTemp : Outport  Port=6
  wires:
  Bus Selector2/3 -> u16_uGDVltg/1  "<u16_uGDVltg>"
  Bus Selector2/2 -> u16_uCtlBrdVltg/1  "<u16_uCtlBrdVltg>"
  Bus Selector2/6 -> u8_tMotoTemp/1  "<u8_tMotoTemp>"
  Bus Selector2/5 -> u8_tPCBTemp/1  "<u8_tPCBTemp>"
  Bus Selector2/4 -> u8_tPwrTubTemp/1  "<u8_tPwrTubTemp>"
  Bus Selector2/1 -> u16_uSplyVltg/1  "<u16_uSplyVltg>"
  busSigIn_SlwTaskOut/1 -> Bus Selector2/1
